simulink library "Kuka_Lib"  (R2026a)
settings: Solver=VariableStepAuto
settings Model: Creator=rosales  LastModifiedBy=rosales

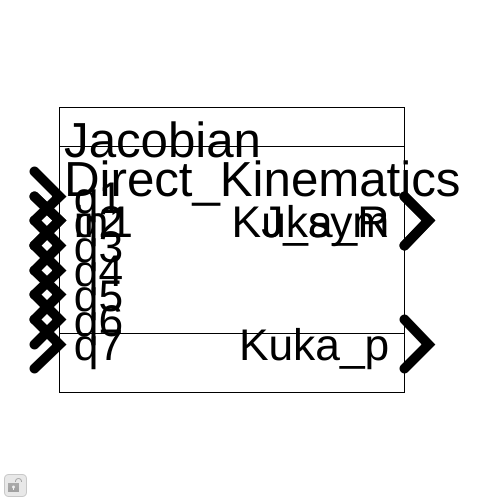
[thumbnail: Simulink's stored preview of the top-level diagram]
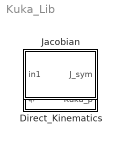
== system Kuka_Lib ==
  Direct_Kinematics : MATLAB Function  TreatAsAtomicUnit=on
  Jacobian : MATLAB Function  TreatAsAtomicUnit=on

== matlab function Kuka_Lib/Jacobian ==
  data: in1 input; J_sym output
function J_sym = jacobian_kuka(in1)
%#codegen

%    This function was generated by the Symbolic Math Toolbox version 26.1.
%    12-May-2026 02:05:02

% in1 = complex(in1);  % if required to enforce complex operations
q1 = in1(1,:);
q2 = in1(2,:);
q3 = in1(3,:);
q4 = in1(4,:);
q5 = in1(5,:);
q6 = in1(6,:);
t2 = cos(q1);
t3 = cos(q2);
t4 = cos(q3);
t5 = cos(q4);
t6 = cos(q5);
t7 = cos(q6);
t8 = sin(q1);
t9 = sin(q2);
t10 = sin(q3);
t11 = sin(q4);
t12 = sin(q5);
t13 = sin(q6);
t14 = t2.*t4;
t15 = t3.*t5;
t16 = t2.*t10;
t17 = t4.*t8;
t18 = t3.*t11;
t19 = t8.*t10;
t20 = t3.*(2.0./5.0);
t21 = t8.*t9.*t11;
t22 = t9.*t10.*t12;
t26 = t2.*t5.*t9;
t27 = t4.*t5.*t9;
t29 = t2.*t9.*t11;
t30 = t5.*t8.*t9;
t31 = t4.*t9.*t11;
t32 = t6.*t9.*t10;
t23 = t3.*t14;
t24 = t3.*t16;
t25 = t3.*t17;
t28 = t3.*t19;
t33 = t15.*(2.0./5.0);
t35 = -t27;
t38 = -t30;
t40 = t26.*(2.0./5.0);
t41 = t30.*(2.0./5.0);
t42 = t31.*(2.0./5.0);
t45 = t15+t31;
t34 = -t23;
t36 = -t28;
t43 = t16+t25;
t44 = t17+t24;
t48 = t18+t35;
t62 = t7.*t45.*(6.3e+1./5.0e+2);
t46 = t14+t36;
t47 = t19+t34;
t49 = t5.*t43;
t50 = t6.*t44;
t51 = t11.*t43;
t52 = t12.*t44;
t55 = t6.*t48;
t58 = t12.*t48;
t53 = t5.*t47;
t54 = t6.*t46;
t56 = t11.*t47;
t57 = t12.*t46;
t59 = t51.*(2.0./5.0);
t63 = t21+t49;
t64 = t38+t51;
t65 = t22+t55;
t60 = -t54;
t61 = t56.*(2.0./5.0);
t66 = t26+t56;
t67 = t6.*t63;
t68 = t12.*t63;
t71 = -t6.*(t29-t53);
t75 = t13.*t65.*(6.3e+1./5.0e+2);
t73 = t7.*t66.*(6.3e+1./5.0e+2);
t76 = t57+t67;
t77 = t52+t71;
t78 = t60+t68;
t82 = t62+t75;
t79 = t13.*t76.*(6.3e+1./5.0e+2);
t81 = t13.*t77.*(6.3e+1./5.0e+2);
t84 = t33+t42+t82;
t83 = -t81;
t85 = t20+t84;
mt1 = [t41-t59+t79+t8.*t9.*(2.0./5.0)+t7.*(t30-t51).*(6.3e+1./5.0e+2),-t40-t61-t73+t81-t2.*t9.*(2.0./5.0),0.0,0.0,0.0,1.0,-t2.*t85,-t8.*t85,t9.*(-2.0./5.0)-t5.*t9.*(2.0./5.0)+t4.*t18.*(2.0./5.0)-t5.*t7.*t9.*(6.3e+1./5.0e+2)+t4.*t7.*t18.*(6.3e+1./5.0e+2)+t3.*t10.*t12.*t13.*(6.3e+1./5.0e+2)-t4.*t6.*t13.*t15.*(6.3e+1./5.0e+2)-t6.*t9.*t11.*t13.*(6.3e+1./5.0e+2),t8,-t2,0.0];
mt2 = [t11.*t17.*(-2.0./5.0)-t16.*t18.*(2.0./5.0)-t7.*t11.*t17.*(6.3e+1./5.0e+2)-t7.*t16.*t18.*(6.3e+1./5.0e+2)-t12.*t13.*t19.*(6.3e+1./5.0e+2)+t12.*t13.*t23.*(6.3e+1./5.0e+2)+t5.*t6.*t13.*t17.*(6.3e+1./5.0e+2)+t6.*t13.*t15.*t16.*(6.3e+1./5.0e+2),t11.*t14.*(2.0./5.0)-t18.*t19.*(2.0./5.0)+t7.*t11.*t14.*(6.3e+1./5.0e+2)+t12.*t13.*t16.*(6.3e+1./5.0e+2)-t7.*t18.*t19.*(6.3e+1./5.0e+2)+t12.*t13.*t25.*(6.3e+1./5.0e+2)-t5.*t6.*t13.*t14.*(6.3e+1./5.0e+2)+t6.*t13.*t15.*t19.*(6.3e+1./5.0e+2),t9.*(t10.*t11.*2.0e+2+t7.*t10.*t11.*6.3e+1-t4.*t12.*t13.*6.3e+1-t5.*t6.*t10.*t13.*6.3e+1).*(-1.0./5.0e+2),-t2.*t9];
mt3 = [-t8.*t9,t3,t46.*t84-t9.*t10.*(t41-t59+t79+t7.*(t30-t51).*(6.3e+1./5.0e+2)),t44.*t84+t9.*t10.*(t40+t61+t73+t83),t18.*(-2.0./5.0)+t27.*(2.0./5.0)-t7.*t18.*(6.3e+1./5.0e+2)+t7.*t27.*(6.3e+1./5.0e+2)+t6.*t13.*t15.*(6.3e+1./5.0e+2)+t6.*t13.*t31.*(6.3e+1./5.0e+2),-t44,t46,-t9.*t10,t13.*(t6.*t17+t6.*t24+t12.*t29-t5.*t12.*t19+t12.*t14.*t15).*(6.3e+1./5.0e+2),t13.*(-t6.*t14+t12.*t21+t6.*t28+t5.*t12.*t16+t12.*t15.*t17).*(6.3e+1./5.0e+2),t13.*(t32-t12.*t18+t12.*t27).*(6.3e+1./5.0e+2),-t66,t64,t45];
mt4 = [(t79+t7.*(t30-t51).*(6.3e+1./5.0e+2)).*(t32-t58)-t82.*(t54-t68),-t82.*(t50+t12.*(t29-t53))-(t73+t83).*(t32-t58),t13.*t15.*(-6.3e+1./5.0e+2)+t7.*t22.*(6.3e+1./5.0e+2)-t13.*t31.*(6.3e+1./5.0e+2)+t6.*t7.*t18.*(6.3e+1./5.0e+2)-t6.*t7.*t27.*(6.3e+1./5.0e+2),t50+t12.*(t29-t53),t78,t32-t58,0.0,0.0,0.0,-t7.*t66+t13.*t77,-t13.*t76-t7.*(t30-t51),t7.*t45+t13.*t65];
J_sym = reshape([mt1,mt2,mt3,mt4],6,7);
end

== matlab function Kuka_Lib/Direct_Kinematics ==
  data: q1 input; Kuka_R output; q2 input; q3 input; q4 input; q5 input; q6 input; q7 input; Kuka_p output
function [Kuka_R,Kuka_p] = direct_kinematics_kuka(q1,q2,q3,q4,q5,q6,q7)
%#codegen

%    This function was generated by the Symbolic Math Toolbox version 26.1.
%    12-May-2026 02:04:17

% q1 = complex(q1);  % if required to enforce complex operations
% q2 = complex(q2);  % if required to enforce complex operations
% q3 = complex(q3);  % if required to enforce complex operations
% q4 = complex(q4);  % if required to enforce complex operations
% q5 = complex(q5);  % if required to enforce complex operations
% q6 = complex(q6);  % if required to enforce complex operations
% q7 = complex(q7);  % if required to enforce complex operations
t2 = cos(q1);
t3 = cos(q2);
t4 = cos(q3);
t5 = cos(q4);
t6 = cos(q5);
t7 = cos(q6);
t8 = cos(q7);
t9 = sin(q1);
t10 = sin(q2);
t11 = sin(q3);
t12 = sin(q4);
t13 = sin(q5);
t14 = sin(q6);
t15 = sin(q7);
t16 = t2.*t4;
t17 = t3.*t5;
t18 = t2.*t11;
t19 = t4.*t9;
t20 = t3.*t12;
t21 = t9.*t11;
t22 = t9.*t10.*t12;
t23 = t10.*t11.*t13;
t27 = t2.*t5.*t10;
t28 = t4.*t5.*t10;
t30 = t2.*t10.*t12;
t31 = t5.*t9.*t10;
t32 = t4.*t10.*t12;
t33 = t6.*t10.*t11;
t24 = t3.*t16;
t25 = t3.*t18;
t26 = t3.*t19;
t29 = t3.*t21;
t35 = -t28;
t42 = t17+t32;
t34 = -t24;
t36 = -t29;
t40 = t18+t26;
t41 = t19+t25;
t45 = t20+t35;
t50 = t14.*t42;
t43 = t16+t36;
t44 = t21+t34;
t46 = t5.*t40;
t47 = t6.*t41;
t48 = t12.*t40;
t49 = t13.*t41;
t54 = t6.*t45;
t57 = t13.*t45;
t51 = t5.*t44;
t52 = t6.*t43;
t55 = t12.*t44;
t56 = t13.*t43;
t60 = t22+t46;
t62 = t23+t54;
t70 = -t14.*(t31-t48);
t63 = t27+t55;
t64 = t6.*t60;
t65 = t13.*t60;
t69 = t7.*t62;
t71 = -t6.*(t30-t51);
t68 = t14.*t63;
t73 = t56+t64;
t74 = t49+t71;
t77 = t7.*t73;
t79 = t7.*t74;
t80 = t70+t77;
t81 = t68+t79;
Kuka_R = reshape([-t15.*(t47+t13.*(t30-t51))-t8.*t81,t8.*t80+t15.*(t52-t65),-t15.*(t33-t57)+t8.*(t50-t69),-t8.*(t47+t13.*(t30-t51))+t15.*t81,-t15.*t80+t8.*(t52-t65),-t8.*(t33-t57)-t15.*(t50-t69),-t7.*t63+t14.*t74,-t14.*t73-t7.*(t31-t48),t7.*t42+t14.*t62],[3,3]);
if nargout > 1
    Kuka_p = [t27.*(-2.0./5.0)-t55.*(2.0./5.0)-t2.*t10.*(2.0./5.0)-t7.*t63.*(6.3e+1./5.0e+2)+t14.*t74.*(6.3e+1./5.0e+2);t31.*(-2.0./5.0)+t48.*(2.0./5.0)-t9.*t10.*(2.0./5.0)-t14.*t73.*(6.3e+1./5.0e+2)-t7.*(t31-t48).*(6.3e+1./5.0e+2);t3.*(2.0./5.0)+t17.*(2.0./5.0)+t32.*(2.0./5.0)+t7.*t42.*(6.3e+1./5.0e+2)+t14.*t62.*(6.3e+1./5.0e+2)];
end
end
